simulink model "untitled"  (R2015a)
settings: Solver=ode45  StartTime=0.0  StopTime=1  RelTol=1e-3
libraries: powerlib x15
settings Model: Creator=MBK  LastModifiedBy=MBK
settings DataIOCC: LimitDataPoints=off

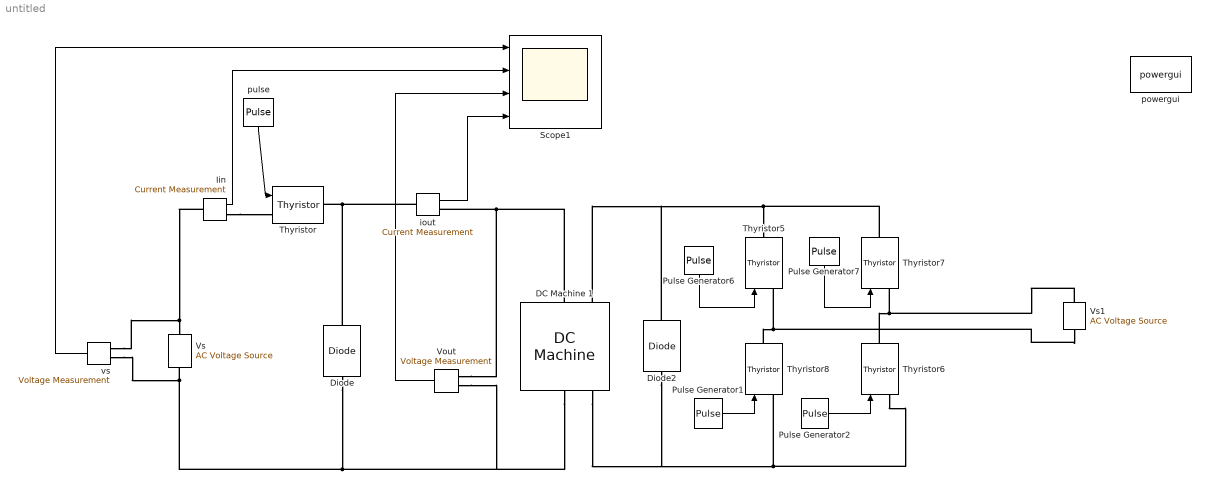
== system untitled ==
  DC Machine 1 : powerlib/Machines/DC Machine  PresetModel=No  MechanicalLoad=Speed w  FieldType=Wound  ShowDetailedParameters=on  MeasurementBus=off  RLa="[ 0.6  0.12]"  RLf="[ 240  120]"  Laf=1.8  MachineConstant=Torque constant (N.m/A)  Ke=1.8  Kt=1.8  J=1  Bm=0  Tf=0  w0=1  Ifinit=1  TsPowergui=0  TsBlock=-1
  "Diode " : powerlib/Power Electronics/Diode  Ron=0.001  Lon=0  Vf=0.8  IC=0  UseSnubber=off  Rs=500  Cs=250e-9  Measurements=off
  Diode2 : powerlib/Power Electronics/Diode  Ron=0.001  Lon=0  Vf=0.8  IC=0  UseSnubber=off  Rs=500  Cs=250e-9  Measurements=off
  "Iin " : powerlib/Measurements/Current Measurement  PhasorSimulation=off  OutputType=Complex  PSBequivalent=0
  Pulse Generator1 : DiscretePulseGenerator  PulseType=Time based  Amplitude=5  Period=0.02  PulseWidth=5  PhaseDelay=240*0.02/360
  Pulse Generator2 : DiscretePulseGenerator  PulseType=Time based  Amplitude=5  Period=0.02  PulseWidth=5  PhaseDelay=60*0.02/360
  Pulse Generator6 : DiscretePulseGenerator  PulseType=Time based  Amplitude=5  Period=0.02  PulseWidth=5  PhaseDelay=60*0.02/360
  Pulse Generator7 : DiscretePulseGenerator  PulseType=Time based  Amplitude=5  Period=0.02  PulseWidth=5  PhaseDelay=240*0.02/360
  Scope1 : Scope  NumInputPorts=4
      settings: YMin=-350~-10~-25~134  YMax=350~150~325~144
  "Thyristor " : powerlib/Power Electronics/Thyristor  Ron=0.001  Lon=0  Vf=0.8  IC=0  Rs=500  Cs=250e-9  Measurements=off
  Thyristor{5..8} (4 alike) : powerlib/Power Electronics/Thyristor  Ron=0.001  Lon=0  Vf=0.8  IC=0  Rs=500  Cs=250e-9  Measurements=off
  "Vout " : powerlib/Measurements/Voltage Measurement  PhasorSimulation=off  OutputType=Complex  PSBequivalent=0
  "Vs  " : powerlib/Electrical Sources/AC Voltage Source  Amplitude=220*sqrt(2)  Phase=0  Frequency=50  SampleTime=0  Measurements=None
  Vs1 : powerlib/Electrical Sources/AC Voltage Source  Amplitude=220*sqrt(2)  Phase=0  Frequency=50  SampleTime=0  Measurements=None
  "iout " : powerlib/Measurements/Current Measurement  PhasorSimulation=off  OutputType=Complex  PSBequivalent=0
  powergui : powerlib/powergui  Priority=1  SimulationMode=Continuous  SolverType=Tustin/Backward Euler (TBE)  SampleTime=50e-6  frequency=60  SPID=off  DisableSnubberDevices=off  DisableRonSwitches=off  DisableVfSwitches=off  SwTol=0  DisplayEquations=off  Interpol=off  methode=off  Ts=100  FunctionMessages=off  echomessages=off  HookPort=off  EnableUseOfTLC=off  x0status=blocks  frequencyindice=0  Pbase=100e6  ErrMax=1e-4  Iterations=50  UnitsV=kV  UnitsW=MW  buscounter=0  RestoreLinks=warning  ResistiveCurrentMeasurement=off  Frange=[0:2:500]  Ylog=off  Xlog=on  ShowGrid=off  save=off  variable=ZData  structure=0  ZoomFFT=off  StartTime=0.0  cycles=1  DisplayStyle=1  fundamental=60  FreqAxis=off  MaxFrequency=1000  frequencyindicesteady=1  RmsSteady=1  display=off
  "pulse " : DiscretePulseGenerator  PulseType=Time based  Period=0.02  PulseWidth=5  PhaseDelay=0.0025
  "vs " : powerlib/Measurements/Voltage Measurement  PhasorSimulation=off  OutputType=Complex  PSBequivalent=0
  wires:
  "pulse "/1 -> "Thyristor "/1
  "vs "/1 -> Scope1/1
  "Iin "/1 -> Scope1/2
  "Vout "/1 -> Scope1/3
  "iout "/1 -> Scope1/4
  Pulse Generator6/1 -> Thyristor5/1
  Pulse Generator7/1 -> Thyristor7/1
  Pulse Generator1/1 -> Thyristor8/1
  Pulse Generator2/1 -> Thyristor6/1
  connections:
  "Diode "/LConn1 -- "Vout "/LConn2 -- DC Machine 1/RConn1 -- "vs "/LConn2 -- "Vs  "/LConn1
  "iout "/LConn1 -- "Diode "/RConn1 -- "Thyristor "/RConn1
  "Vout "/LConn1 -- DC Machine 1/LConn1 -- "iout "/RConn1
  "Iin "/RConn1 -- "Thyristor "/LConn1
  "Iin "/LConn1 -- "vs "/LConn1 -- "Vs  "/RConn1
  Vs1/RConn1 -- Thyristor6/RConn1 -- Thyristor7/LConn1
  Vs1/LConn1 -- Thyristor8/RConn1 -- Thyristor5/LConn1
  Thyristor6/LConn1 -- DC Machine 1/RConn2 -- Diode2/LConn1 -- Thyristor8/LConn1
  Thyristor7/RConn1 -- Diode2/RConn1 -- DC Machine 1/LConn2 -- Thyristor5/RConn1
